simulink model "first_model_simulink"  (R2023a)
settings: Solver=VariableStepAuto  StartTime=0.0  StopTime=sim_time  MaxStep=1  RelTol=1e-3
values from neighbouring files (symbols this model uses):
  A_f = 2    [parameter_definiciton.m]
  air_dens = 1.22521    [parameter_definiciton.m]
  angle_road = atan(slope_road/100)    [parameter_definiciton.m]
  C_d = 0.35    [parameter_definiciton.m]
  f_r = 0.017    [parameter_definiciton.m]
  g = 9.8    [parameter_definiciton.m]
  m_v = 1000    [parameter_definiciton.m]
  wind_speed = 0    [parameter_definiciton.m]
libraries: simulink x2
settings Model: Creator=citcea  LastModifiedBy=citcea

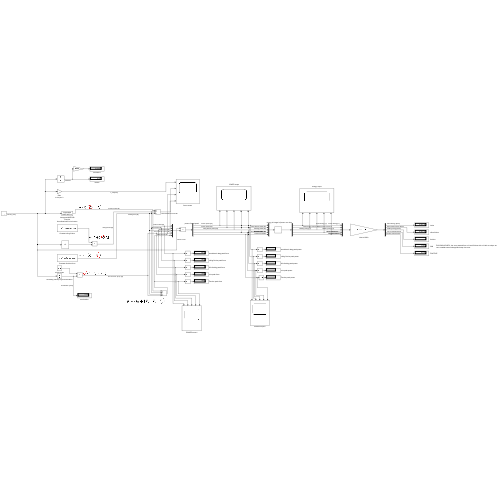
[thumbnail: Simulink's stored preview of the top-level diagram]
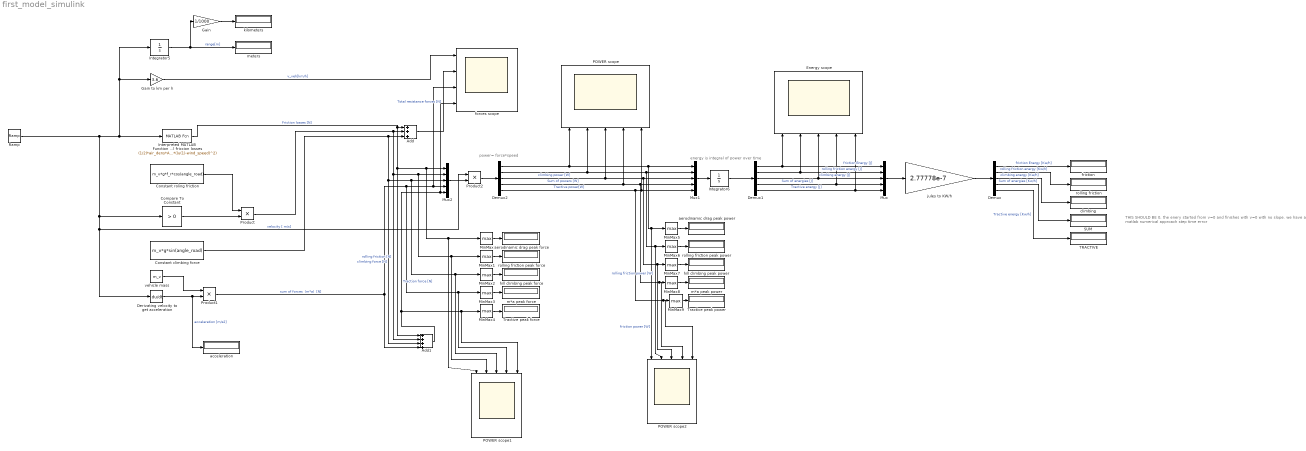
== system first_model_simulink ==
  note: energy is integral of power over time
  note: THIS SHOULD BE 0, the enery started from v=0 and finishes with v=0 with no slope. we have a matlab numerical approach step time error
  note: power= force*speed
  Add : Sum  Inputs=+++
  Add1 : Sum  Inputs=++++
  Compare To Constant : simulink/Logic and Bit Operations/Compare To Constant  relop=>  const=0  OutDataTypeStr=boolean
  Constant climbing force : Constant  Value=m_v*g*sin(angle_road)
  Constant roling friction : Constant  Value=m_v*g*f_r*cos(angle_road)
  Demux : Demux  Outputs=5
  Demux1 : Demux  Outputs=5
  Demux2 : Demux  Outputs=5
  Derivating velocity to get acceleration : Derivative
  Energy scope : Scope  NumInputPorts=5
  Gain : Gain  Gain=1/1000
  Gain to km per h : Gain  Gain=3.6
  Integrator5 : Integrator
  Integrator6 : Integrator
  Interpreted MATLAB Function Aerodinamical friccion losses : MATLABFcn  MATLABFcn=(1/2)*air_dens*A_f*C_d*((u(1)-wind_speed)^2)
  MinMax{,1..9} (10 alike) : MinMax  Function=max
  Mux : Mux  Inputs=5
  Mux1 : Mux  Inputs=5
  Mux2 : Mux  Inputs=5
  POWER scope : Scope  NumInputPorts=5
  POWER scope1 : Scope  NumInputPorts=5
  POWER scope2 : Scope  NumInputPorts=5
  Product : Product
  Product1 : Product
  Product2 : Product
  Ramp : simulink/Sources/Ramp  slope=(100/3.6)/5.9  start=0  InitialOutput=0
  "SUM " : Display
  TRACTIVE : Display
  Tractive peak force : Display
  Tractive peak power : Display
  acceleration : Display
  aerodinamic drag peak force : Display
  aerodinamic drag peak power : Display
  climbing : Display
  forces scope : Scope  NumInputPorts=4
  friction : Display
  hill climbing peak force : Display
  hill climbing peak power : Display
  jules to KW/h : Gain  Gain=2.77778e-7
  kilometers : Display
  m*a peak force : Display
  m*a peak power : Display
  meters : Display
  "rolling friction " : Display
  rolling friction peak force : Display
  rolling friction peak power : Display
  vehicle mass : Constant  Value=m_v
  wires:
  Interpreted MATLAB Function Aerodinamical friccion losses/1 -> Add1/1, MinMax/1, POWER scope1/1, Mux2/1, Add/1  "Friction losses [N]"
  Gain to km per h/1 -> forces scope/1  "v_veh[km/h]"
  Compare To Constant/1 -> Product/2
  Constant roling friction/1 -> Product/1
  Product/1 -> Add1/2, Mux2/2, MinMax1/1, POWER scope1/2, Add/2  "rolling friction [N]"
  Constant climbing force/1 -> Add1/3, POWER scope1/3, MinMax2/1, Mux2/3, Add/3  "climbing force [N]"
  Add/1 -> forces scope/2  "Total resistance forces [N]"
  vehicle mass/1 -> Product1/1
  Derivating velocity to get acceleration/1 -> acceleration/1, Product1/2  "acceleration [m/s2]"
  Product1/1 -> POWER scope1/4, MinMax3/1, Mux2/4, forces scope/3, Add1/4  "sum of forces  (m*a)  [N]"
  Add1/1 -> forces scope/4, Mux2/5, POWER scope1/5, MinMax4/1  "Traction force [N]"
  Ramp/1 -> Derivating velocity to get acceleration/1, Product2/1, Compare To Constant/1, Integrator5/1, Gain to km per h/1, Interpreted MATLAB Function Aerodinamical friccion losses/1  "velocity [ m/s]"
  Demux2/1 -> POWER scope2/1, MinMax5/1, Mux1/1, POWER scope/1  "friction power [W]"
  Demux2/3 -> MinMax7/1, POWER scope2/3, Mux1/3, POWER scope/3  "climbing power [W]"
  Demux2/4 -> POWER scope2/4, MinMax8/1, Mux1/4, POWER scope/4  "Sum of powers [W]"
  Demux2/2 -> MinMax6/1, POWER scope2/2, Mux1/2, POWER scope/2  "rolling friction power [W]"
  Demux2/5 -> POWER scope2/5, MinMax9/1, Mux1/5, POWER scope/5  "Tractive power[W]"
  Demux1/1 -> Mux/1, Energy scope/1  "friction Energy [J]"
  Demux1/2 -> Mux/2, Energy scope/2  "rolling friction energy [J]"
  Demux1/3 -> Mux/3, Energy scope/3  "climbing energy [J]"
  Demux1/4 -> Mux/4, Energy scope/4  "Sum of energies [J]"
  Demux1/5 -> Mux/5, Energy scope/5  "Tractive energy [J]"
  Integrator5/1 -> Gain/1, meters/1  "range[m]"
  Gain/1 -> kilometers/1
  Mux/1 -> jules to KW/h/1
  jules to KW/h/1 -> Demux/1
  Demux/1 -> friction/1  "friction Energy [Kw/h]"
  Demux/2 -> "rolling friction "/1  "rolling friction energy [Kw/h]"
  Demux/3 -> climbing/1  "climbing energy [Kw/h]"
  Demux/4 -> "SUM "/1  "Sum of energies [Kw/h]"
  Demux/5 -> TRACTIVE/1  "Tractive energy [Kw/h]"
  Mux1/1 -> Integrator6/1
  Integrator6/1 -> Demux1/1
  Mux2/1 -> Product2/2
  Product2/1 -> Demux2/1
  MinMax/1 -> aerodinamic drag peak force/1
  MinMax1/1 -> rolling friction peak force/1
  MinMax2/1 -> hill climbing peak force/1
  MinMax3/1 -> m*a peak force/1
  MinMax4/1 -> Tractive peak force/1
  MinMax7/1 -> hill climbing peak power/1
  MinMax5/1 -> aerodinamic drag peak power/1
  MinMax6/1 -> rolling friction peak power/1
  MinMax8/1 -> m*a peak power/1
  MinMax9/1 -> Tractive peak power/1
